simulink model "PMSM_Hall_model"  (R2025b)
settings: Solver=VariableStepAuto  StartTime=0.0  StopTime=10.0  RelTol=1e-3
values from neighbouring files (symbols this model uses):
  B = 0.0025    [PMSM_Hall_Model_script.m]
  Damping_viscous = 0.00012    [PMSM_Hall_Model_script.m]
  J = 4.5e-5    (= 4.5e-05)    [PMSM_Hall_Model_script.m]
  Ki_Id = omg_clc * R_s    (= 464.72)    [PMSM_Hall_Model_script.m]
  Ki_Iq = omg_clc * R_s    (= 464.72)    [PMSM_Hall_Model_script.m]
  Kp_Id = omg_clc * Ld    (= 22.608)    [PMSM_Hall_Model_script.m]
  Kp_Iq = omg_clc * Lq    (= 22.608)    [PMSM_Hall_Model_script.m]
  motor_polepairs = 7    [PMSM_Hall_Model_script.m]
  pwm_frequency = 20e3    (= 20000)    [PMSM_Hall_Model_script.m]
  x = 600    [PMSM_Hall_Model_script.m]
libraries: nesl_utility x9, slpidlib x5, fl_lib x5, mcbeeMathTransformLib x3, ee_lib x3, mcbcontrolslib x1, mcbsensorlessestimatorlib x1, mcbplantlib x1, autolibpmsmexterior x1, sdl_lib x1
settings Model: Creator=Surinova  LastModifiedBy=Surinova

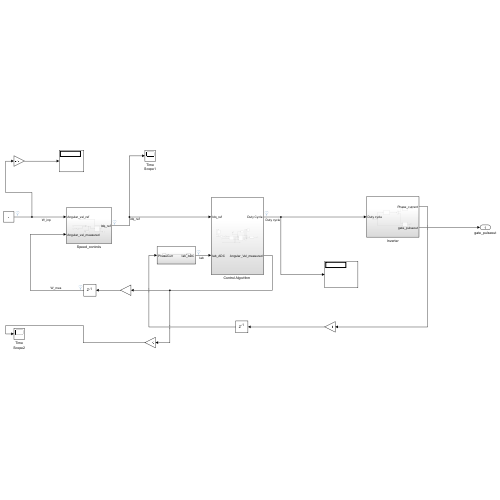
[thumbnail: Simulink's stored preview of the top-level diagram]
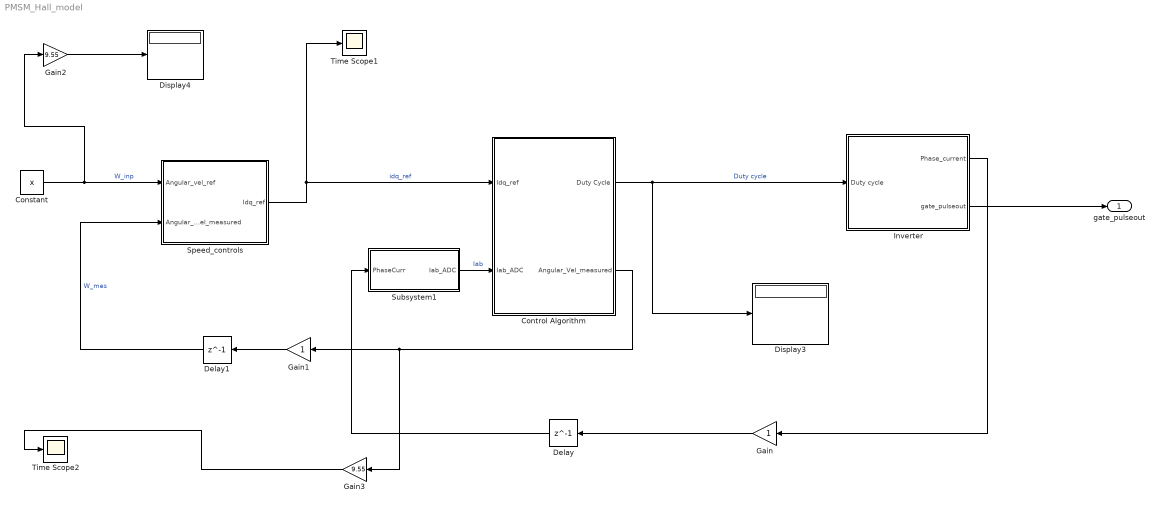
== system PMSM_Hall_model ==
  Constant : Constant  Value=x
  "Control Algorithm " : Subsystem
  Delay : Delay  DelayLength=1
  Delay1 : Delay  DelayLength=1
  Display3 : Display
  Display4 : Display
  Gain : Gain
  Gain1 : Gain
  Gain2 : Gain  Gain=9.55
  Gain3 : Gain  Gain=9.55
  Inverter : Subsystem
  Speed_controls : Subsystem
  Subsystem1 : Subsystem
  Time Scope1 : Scope
      settings: TimeUnits=Metric (based on Time Span)  ActiveDisplayYMinimum=-1278.396312713623  ActiveDisplayYMaximum=607.25992965698242  YLabel=Amplitude
  Time Scope2 : Scope
      settings: TimeUnits=Metric (based on Time Span)  ActiveDisplayYMinimum=-2551.3535904439232  ActiveDisplayYMaximum=7986.0366937033405  YLabel=Amplitude  DataLoggingVariableName=ScopeData5
  gate_pulseout : Outport
  wires:
  Speed_controls/1(Idq_ref) -> Time Scope1/1, "Control Algorithm "/1(Idq_ref)  "idq_ref"
  Delay/1 -> Subsystem1/1(PhaseCurr)
  "Control Algorithm "/2(Angular_Vel_measured) -> Gain1/1, Gain3/1
  Gain/1 -> Delay/1
  Delay1/1 -> Speed_controls/2(Angular_vel_measured)  "W_mes"
  Constant/1 -> Gain2/1, Speed_controls/1(Angular_vel_ref)  "W_inp"
  Subsystem1/1(Iab_ADC) -> "Control Algorithm "/2(Iab_ADC)  "Iab"
  Gain3/1 -> Time Scope2/1
  "Control Algorithm "/1(Duty Cycle) -> Inverter/1(Duty cycle), Display3/1  "Duty cycle"
  Inverter/1(Phase_current) -> Gain/1
  Gain2/1 -> Display4/1
  Inverter/2(gate_pulseout) -> gate_pulseout/1
  Gain1/1 -> Delay1/1

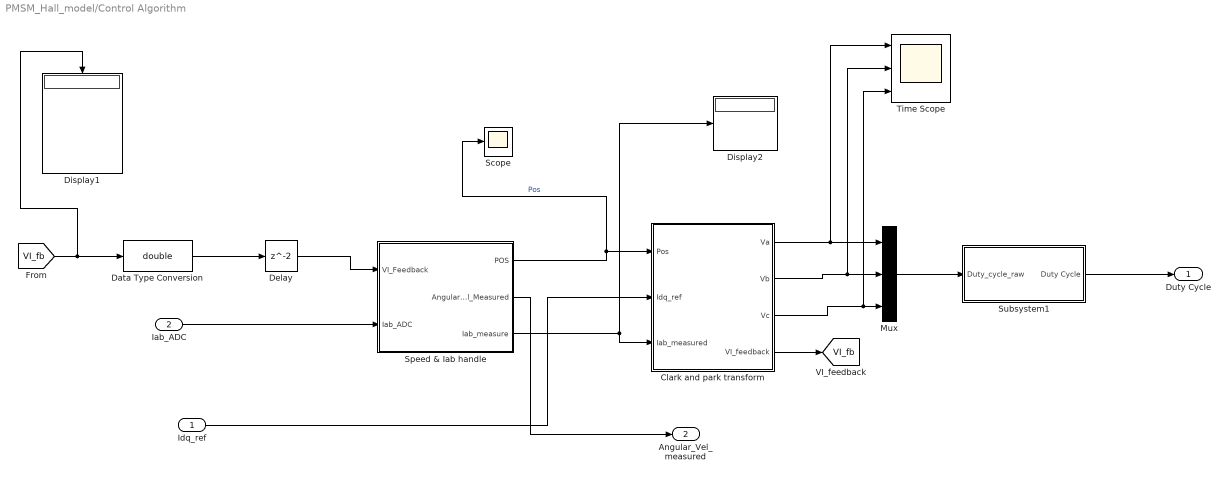
== system PMSM_Hall_model/Control Algorithm  ==
  Idq_ref : Inport
  Iab_ADC : Inport  Port=2
  Clark and park transform : Subsystem
  Data Type Conversion : DataTypeConversion  OutDataTypeStr=double  SaturateOnIntegerOverflow=off  RndMeth=Floor
  Delay : Delay
  Display1 : Display
  Display2 : Display
  Mux : Mux  Inputs=3
  Scope : Scope
      settings: ActiveDisplayYMinimum=-2.9858848726720835  ActiveDisplayYMaximum=10.141823403799465  DataLoggingVariableName=ScopeData4
  Speed & Iab handle : Subsystem
  Subsystem1 : Subsystem
  Time Scope : Scope  NumInputPorts=3
      settings: TimeUnits=Metric (based on Time Span)  ActiveDisplayYMinimum=-2.8960393222402327  ActiveDisplayYMaximum=4.8327650583252995  YLabel=Amplitude  DataLoggingVariableName=ScopeData2
  Duty Cycle : Outport
  Angular_Vel_measured : Outport  Port=2
  tag scope: VI_fb=global
  wires:
  Clark and park transform/4(VI_feedback) -> [VI_fb]
  Clark and park transform/3(Vc) -> Mux/3, Time Scope/3
  [VI_fb] -> Display1/1, Data Type Conversion/1
  Mux/1 -> Subsystem1/1(Duty_cycle_raw)
  Iab_ADC/1 -> Speed & Iab handle/2(Iab_ADC)
  Speed & Iab handle/3(Iab_measure) -> Clark and park transform/3(Iab_measured), Display2/1
  Clark and park transform/2(Vb) -> Mux/2, Time Scope/2
  Clark and park transform/1(Va) -> Time Scope/1, Mux/1
  Speed & Iab handle/2(Angular_Vel_Measured) -> Angular_Vel_measured/1
  Idq_ref/1 -> Clark and park transform/2(Idq_ref)
  Delay/1 -> Speed & Iab handle/1(VI_Feedback)
  Data Type Conversion/1 -> Delay/1
  Speed & Iab handle/1(POS) -> Scope/1, Clark and park transform/1(Pos)  "Pos"
  Subsystem1/1(Duty Cycle) -> Duty Cycle/1

== system PMSM_Hall_model/Inverter ==
  Duty cycle : Inport
  Codegen : Subsystem
  Simulation : Subsystem
  Subsystem2 : Subsystem
  Variant Sink : VariantSink  VariantControlMode=sim codegen switching  ShowConditionOnBlock=on  VariantControls={(codegen), (sim)}
  Phase_current : Outport
  gate_pulseout : Outport  Port=2
  wires:
  Duty cycle/1 -> Simulation/2(Duty_cycle), Subsystem2/1(Duty cycle)
  Subsystem2/1(Duty_cycle_6pulse) -> Variant Sink/1  "Gate_pulse"
  Simulation/1(Phase_current) -> Phase_current/1
  Variant Sink/2 -> Simulation/1(Gate_pulse)
  Variant Sink/1 -> Codegen/1(gate_pulse)
  Codegen/1(gate_pulseout) -> gate_pulseout/1

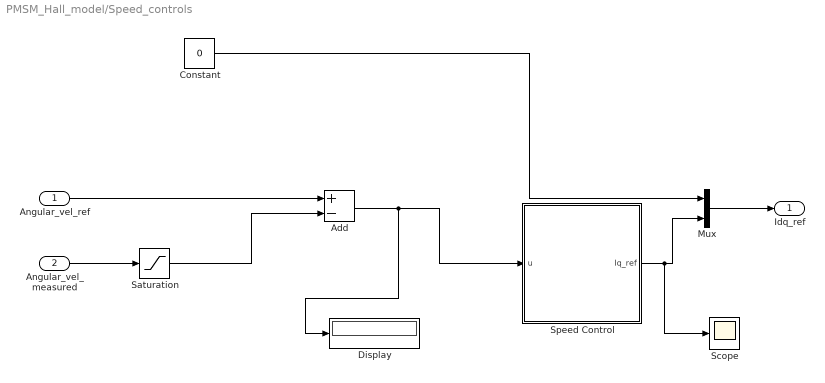
== system PMSM_Hall_model/Speed_controls ==
  Angular_vel_ref : Inport
  Angular_vel_measured : Inport  Port=2
  Add : Sum  Inputs=+-
  Constant : Constant  Value=0
  Display : Display
  Mux : Mux  Inputs=2
  Saturation : Saturate  UpperLimit=600  LowerLimit=-600
  Scope : Scope
      settings: ActiveDisplayYMinimum=-1  ActiveDisplayYMaximum=1  DataLoggingVariableName=ScopeData3
  Speed Control : Subsystem
  Idq_ref : Outport  PortDimensions=2
  wires:
  Angular_vel_measured/1 -> Saturation/1
  Add/1 -> Display/1, Speed Control/1(u)
  Mux/1 -> Idq_ref/1
  Speed Control/1(Iq_ref) -> Scope/1, Mux/2
  Constant/1 -> Mux/1
  Angular_vel_ref/1 -> Add/1
  Saturation/1 -> Add/2

== system PMSM_Hall_model/Subsystem1 ==
  PhaseCurr : Inport
  Iab_ADC : Outport
  wires:
  PhaseCurr/1 -> Iab_ADC/1

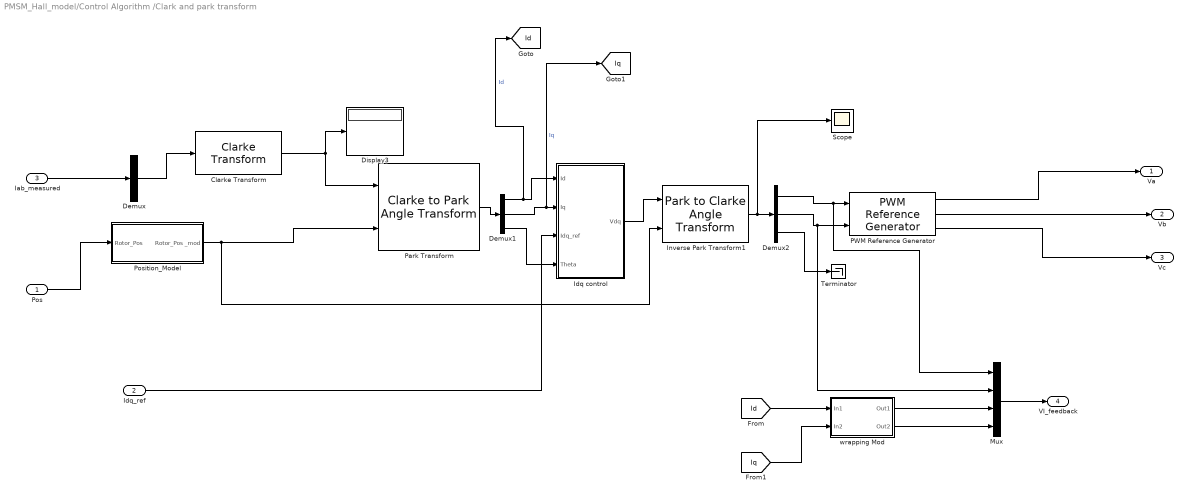
== system PMSM_Hall_model/Control Algorithm /Clark and park transform ==
  Pos : Inport
  Idq_ref : Inport  Port=2
  Iab_measured : Inport  Port=3
  Clarke Transform : mcbeeMathTransformLib/Clarke Transform  VariantControl=Variant2  PowerInvariant=off  UseWithEmbedded=on  PhaseInput=Three inputs
      settings: LibrarySourceBlock=mcblib/Controls/Math Transforms/Clarke Transform
  Demux : Demux  Outputs=1
  Demux1 : Demux  Outputs=3
  Demux2 : Demux  Outputs=3
  Display3 : Display
  Idq control : Subsystem
  Inverse Park Transform1 : mcbeeMathTransformLib/Park to Clarke Angle Transform  AxisAlignment=D-axis  UseWithEmbedded=on  PhaseInput=Three inputs  ThetaInput=Electrical position  AngleInput=Radians  N_points=1024
      settings: LibrarySourceBlock=mcbhdllib/Controls/Math Transforms/Inverse Park Transform
  Mux : Mux
  PWM Reference Generator : mcbcontrolslib/PWM Reference Generator  inSignal=Valphabeta  modType=SVM: space vector modulation
      settings: LibrarySourceBlock=mcbhdllib/Controls/Math Transforms/PWM Reference Generator
  Park Transform : mcbeeMathTransformLib/Clarke to Park Angle Transform  AxisAlignment=D-axis  UseWithEmbedded=on  PhaseInput=Three inputs  ThetaInput=Electrical position  AngleInput=Radians  N_points=1024
      settings: LibrarySourceBlock=mcblib/Controls/Math Transforms/Park Transform
  Position_Model : Subsystem
  Scope : Scope
      settings: ActiveDisplayYMinimum=-1.6231207105132253  ActiveDisplayYMaximum=1.9168476700347847  DataLoggingVariableName=ScopeData9
  Terminator : Terminator
  wrapping Mod : Subsystem
  Va : Outport
  Vb : Outport  Port=2
  Vc : Outport  Port=3
  VI_feedback : Outport  Port=4
  tag scope: Id=global, Iq=global
  wires:
  Clarke Transform/1 -> Park Transform/1, Display3/1
  Demux/1 -> Clarke Transform/1
  PWM Reference Generator/1 -> Va/1
  PWM Reference Generator/2 -> Vb/1
  PWM Reference Generator/3 -> Vc/1
  Idq_ref/1 -> Idq control/3(Idq_ref)
  Mux/1 -> VI_feedback/1
  Iab_measured/1 -> Demux/1
  wrapping Mod/1(Out1) -> Mux/3
  wrapping Mod/2(Out2) -> Mux/4
  Pos/1 -> Position_Model/1(Rotor_Pos)
  Position_Model/1(Rotor_Pos _mod) -> Inverse Park Transform1/2, Park Transform/2
  Park Transform/1 -> Demux1/1
  Demux1/2 -> [Iq], Idq control/2(Iq)  "Iq"
  Demux1/3 -> Idq control/4(Theta)
  Idq control/1(Vdq) -> Inverse Park Transform1/1
  Inverse Park Transform1/1 -> Scope/1, Demux2/1
  Demux2/1 -> Mux/1, PWM Reference Generator/1
  Demux2/2 -> Mux/2, PWM Reference Generator/2
  Demux2/3 -> Terminator/1
  Demux1/1 -> [Id], Idq control/1(Id)  "Id"
  [Id] -> wrapping Mod/1(In1)
  [Iq] -> wrapping Mod/2(In2)

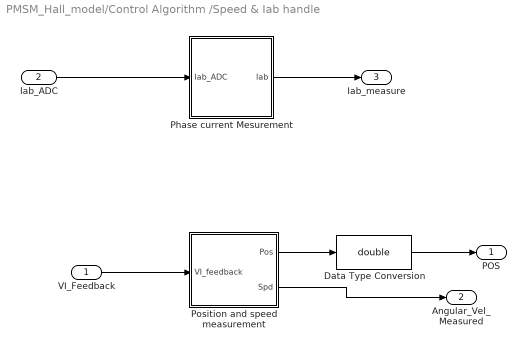
== system PMSM_Hall_model/Control Algorithm /Speed & Iab handle ==
  VI_Feedback : Inport
  Iab_ADC : Inport  Port=2
  Data Type Conversion : DataTypeConversion  OutDataTypeStr=double  SaturateOnIntegerOverflow=off  RndMeth=Floor
  Phase current Mesurement : Subsystem
  Position and speed measurement : Subsystem
  POS : Outport
  Angular_Vel_Measured : Outport  Port=2
  Iab_measure : Outport  Port=3
  wires:
  VI_Feedback/1 -> Position and speed measurement/1(VI_feedback)
  Position and speed measurement/1(Pos) -> Data Type Conversion/1
  Position and speed measurement/2(Spd) -> Angular_Vel_Measured/1
  Iab_ADC/1 -> Phase current Mesurement/1(Iab_ADC)
  Phase current Mesurement/1(Iab) -> Iab_measure/1
  Data Type Conversion/1 -> POS/1

== system PMSM_Hall_model/Control Algorithm /Subsystem1 ==
  Duty_cycle_raw : Inport
  Add : Sum
  Constant : Constant  Value=1.45
  Gain : Gain  Gain=1/3
  Duty Cycle : Outport
  wires:
  Constant/1 -> Add/2
  Add/1 -> Gain/1
  Duty_cycle_raw/1 -> Add/1
  Gain/1 -> Duty Cycle/1

== system PMSM_Hall_model/Inverter/Codegen ==
  note: Hardware region
      | gate pulse fed todriver via controller
  gate_pulse : Inport
  gate_pulseout : Outport
  wires:
  gate_pulse/1 -> gate_pulseout/1

== system PMSM_Hall_model/Inverter/Simulation ==
  Gate_pulse : Inport
  Duty_cycle : Inport  Port=2
  Inverter&motor_Plant_model : Subsystem
  Scope : Scope  NumInputPorts=2
      settings: ActiveDisplayYMinimum=-225.10774527747819  ActiveDisplayYMaximum=225.10294010409339  DataLoggingVariableName=ScopeData7
  Simscape_Plantmodel : Subsystem
  Time Scope : Scope
      settings: TimeUnits=Metric (based on Time Span)  ActiveDisplayYMinimum=-4.9999999999993694  ActiveDisplayYMaximum=44.999999999994344  YLabel=Amplitude
  Phase_current : Outport
  wires:
  Inverter&motor_Plant_model/1(Electrical Pos) -> Scope/1  "Ele_Pos"
  Simscape_Plantmodel/1(Angular_vel_measured) -> Time Scope/1  "W_fb_sim"
  Inverter&motor_Plant_model/3(Motor_trq) -> Scope/2  "Motor_rpm"
  Inverter&motor_Plant_model/2(PhaseCurrent) -> Phase_current/1  "Phase_current"
  Gate_pulse/1 -> Simscape_Plantmodel/1(Duty Cycle_6pulse)
  Duty_cycle/1 -> Inverter&motor_Plant_model/1(Duty_cycle)

== system PMSM_Hall_model/Inverter/Subsystem2 ==
  Duty cycle : Inport
  Demux : Demux  Outputs=3
  Demux1 : Demux  Outputs=3
  Gate_pulse : Scope  NumInputPorts=6
      settings: TimeUnits=Metric (based on Time Span)  ActiveDisplayYMinimum=-0.2043367875881458  ActiveDisplayYMaximum=0.55931759444230922  YLabel=Amplitude  DataLoggingVariableName=ScopeData10
  Mux : Mux  Inputs=6
  Subsystem : Subsystem
  Duty_cycle_6pulse : Outport
  wires:
  Demux1/1 -> Mux/2, Gate_pulse/4  "GA_L"
  Demux/2 -> Mux/3, Gate_pulse/2  "GB_H"
  Duty cycle/1 -> Demux/1, Subsystem/1(Duty Cycle)
  Demux/1 -> Mux/1, Gate_pulse/1  "GA_H"
  Subsystem/1(Gate_Lowside) -> Demux1/1
  Demux1/2 -> Mux/4, Gate_pulse/5  "GB_L"
  Demux1/3 -> Mux/6, Gate_pulse/6  "GC_L"
  Demux/3 -> Mux/5, Gate_pulse/3  "GC_H"
  Mux/1 -> Duty_cycle_6pulse/1

== system PMSM_Hall_model/Speed_controls/Speed Control ==
  u : Inport
  PID Controller : slpidlib/PID Controller  Controller=PI  Form=Parallel  TimeDomain=Continuous-time  UseExternalTs=off  SampleTime=-1  IntegratorMethod=Forward Euler  FilterMethod=Forward Euler  ControllerParametersSource=internal  P=1  I=0  UseKiTs=off  D=0  UseExternalDerivativeSource=off  N=100  UseFilter=on  TunerSelectOption=Transfer Function Based (PID Tuner App)  InitialConditionSource=internal  InitialConditionForIntegrator=0  InitialConditionForFilter=0  DifferentiatorICPrevScaledInput=0  ExternalReset=none  TrackingMode=off  Kt=1  LimitOutput=off  SatLimitsSource=internal  UpperSaturationLimit=inf  LowerSaturationLimit=-inf  LinearizeAsGain=on  AntiWindupMode=none  Kb=1  LimitIntegrator=off  UpperIntegratorSaturationLimit=inf  LowerIntegratorSaturationLimit=-inf  POutMin=[]  POutMax=[]  IOutMin=[]  IOutMax=[]  DOutMin=[]  DOutMax=[]  NOutMin=[]  NOutMax=[]  SumOutMin=[]  SumOutMax=[]  SaturationOutMin=[]  SaturationOutMax=[]  PParamMin=[]  PParamMax=[]  IParamMin=[]  IParamMax=[]  DParamMin=[]  DParamMax=[]  NParamMin=[]  NParamMax=[]  KbParamMin=[]  KbParamMax=[]  KtParamMin=[]  KtParamMax=[]  KbOutMin=[]  KbOutMax=[]  KtOutMin=[]  KtOutMax=[]  IntegratorOutMin=[]  IntegratorOutMax=[]  FilterOutMin=[]  FilterOutMax=[]  SumI1OutMin=[]  SumI1OutMax=[]  SumI2OutMin=[]  SumI2OutMax=[]  SumI3OutMin=[]  SumI3OutMax=[]  SumI4OutMin=[]  SumI4OutMax=[]  SumDOutMin=[]  SumDOutMax=[]  DifferentiatorOutMin=[]  DifferentiatorOutMax=[]  FilterDiffOutCoefMin=[]  FilterDiffOutCoefMax=[]  ReciprocalOutMin=[]  ReciprocalOutMax=[]  SumDenOutMin=[]  SumDenOutMax=[]  SumNumOutMin=[]  SumNumOutMax=[]  DivideOutMin=[]  DivideOutMax=[]  UdiffTsProdOutMin=[]  UdiffTsProdOutMax=[]  NTsProdOutMin=[]  NTsProdOutMax=[]  UintegralTsProdOutMin=[]  UintegralTsProdOutMax=[]  UngainTsProdOutMin=[]  UngainTsProdOutMax=[]  ClampingZeroOutDataTypeStr=Inherit: Inherit via back propagation  ClampingZeroOutMin=[]  ClampingZeroOutMax=[]  FilterDenConstantOutDataTypeStr=Inherit: Inherit via back propagation  FilterDenConstantOutMin=[]  FilterDenConstantOutMax=[]  PCopyOutDataTypeStr=Inherit: Inherit via back propagation  PCopyOutMin=[]  PCopyOutMax=[]  NCopyOutDataTypeStr=Inherit: Inherit via back propagation  NCopyOutMin=[]  NCopyOutMax=[]  IntegratorContinuousStateAttributes=''  IntegratorStateMustResolveToSignalObject=off  IntegratorRTWStateStorageClass=Auto  FilterContinuousStateAttributes=''  FilterStateMustResolveToSignalObject=off  FilterRTWStateStorageClass=Auto  ParallelPVariant=InternalParameters  IdealPVariant=Disabled  IVariant=InternalParameters  DVariant=Disabled  IntegratorVariant=Continuous  SatVariant=Disabled  AWVariant=Passthrough  PCopyVariant=Disabled  TRVariant=Disabled  FdbkBlocksVariant=Forward  IdealPFdbkVariant=Disabled  SatFdbkVariant=Disabled  DerivativeFilterVariant=Disabled  NVariant=Disabled  NCopyVariant=Disabled_SignalSpec  FilterICVariant=Disabled  IntegratorICVariant=InternalICs  ExternalResetVariant=Disabled  TRSumVariant=Passthrough  SumFdbkVariant=Disabled  SumVariant=Sum_PI  TsampFilterVariant=InternalTs  TsampNgainVariant=Passthrough  TsampIntegralVariant=Disabled_SignalSpec  ExternalSaturationOutDataTypeStr=Inherit: Same as second input  DerivativeSourceVariant=Disabled  PreIntVariant=InternalPreInt
  Iq_ref : Outport
  wires:
  u/1 -> PID Controller/1
  PID Controller/1 -> Iq_ref/1

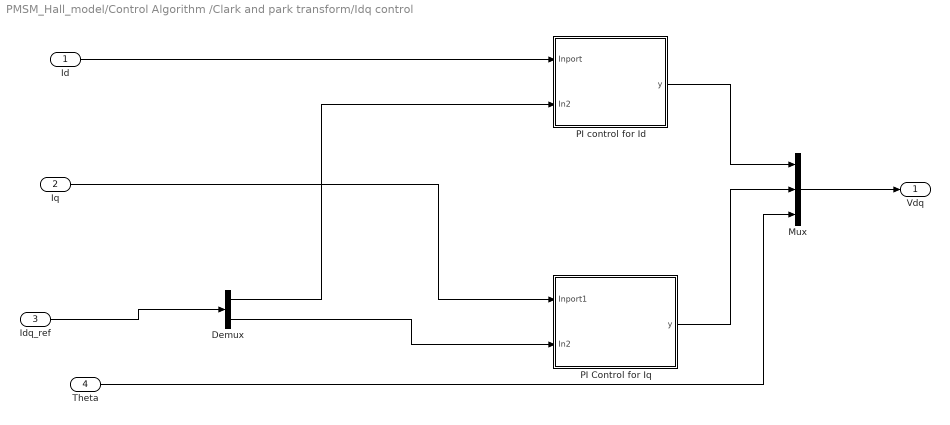
== system PMSM_Hall_model/Control Algorithm /Clark and park transform/Idq control ==
  Id : Inport
  Iq : Inport  Port=2
  Idq_ref : Inport  Port=3
  Theta : Inport  Port=4
  Demux : Demux  Outputs=2
  Mux : Mux  Inputs=3
  PI Control for Iq : Subsystem
  PI control for Id : Subsystem
  Vdq : Outport
  wires:
  Idq_ref/1 -> Demux/1
  Id/1 -> PI control for Id/1(Inport)
  Iq/1 -> PI Control for Iq/1(Inport1)
  Demux/1 -> PI control for Id/2(In2)
  Demux/2 -> PI Control for Iq/2(In2)
  PI control for Id/1(y) -> Mux/1
  PI Control for Iq/1(y) -> Mux/2
  Mux/1 -> Vdq/1
  Theta/1 -> Mux/3

== system PMSM_Hall_model/Control Algorithm /Clark and park transform/Position_Model ==
  Rotor_Pos : Inport
  Constant : Constant  Value=2*3.141
  Data Type Conversion1 : DataTypeConversion  OutDataTypeStr=double  ConvertRealWorld=Stored Integer (SI)  RndMeth=Floor
  Display : Display
  Mod : Math  Operator=mod
  Rotor_Pos _mod : Outport
  wires:
  Mod/1 -> Data Type Conversion1/1
  Constant/1 -> Mod/2
  Rotor_Pos/1 -> Mod/1  "Eps"
  Data Type Conversion1/1 -> Rotor_Pos _mod/1, Display/1

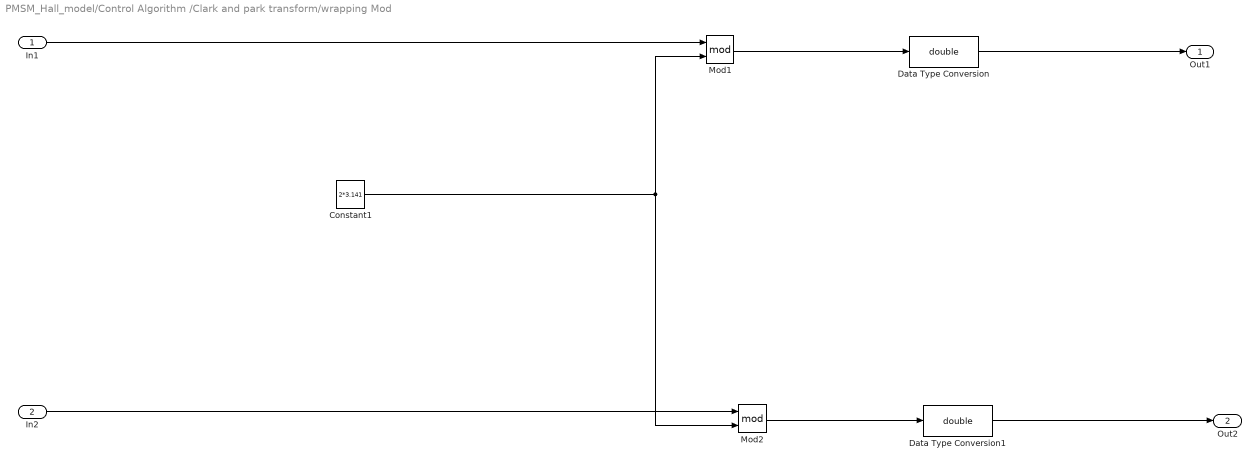
== system PMSM_Hall_model/Control Algorithm /Clark and park transform/wrapping Mod ==
  In1 : Inport
  In2 : Inport  Port=2
  Constant1 : Constant  Value=2*3.141
  Data Type Conversion : DataTypeConversion  OutDataTypeStr=double  SaturateOnIntegerOverflow=off  RndMeth=Floor
  Data Type Conversion1 : DataTypeConversion  OutDataTypeStr=double  SaturateOnIntegerOverflow=off  RndMeth=Floor
  Mod1 : Math  Operator=mod
  Mod2 : Math  Operator=mod
  Out1 : Outport
  Out2 : Outport  Port=2
  wires:
  Constant1/1 -> Mod2/2, Mod1/2
  In1/1 -> Mod1/1
  In2/1 -> Mod2/1
  Mod2/1 -> Data Type Conversion1/1
  Mod1/1 -> Data Type Conversion/1
  Data Type Conversion/1 -> Out1/1
  Data Type Conversion1/1 -> Out2/1

== system PMSM_Hall_model/Control Algorithm /Speed & Iab handle/Phase current Mesurement ==
  Iab_ADC : Inport
  Data Type Conversion : DataTypeConversion  SaturateOnIntegerOverflow=off  RndMeth=Floor
  Iab : Outport
  wires:
  Data Type Conversion/1 -> Iab/1
  Iab_ADC/1 -> Data Type Conversion/1

== system PMSM_Hall_model/Control Algorithm /Speed & Iab handle/Position and speed measurement ==
  VI_feedback : Inport
  Demux : Demux
  Extended EMF Observer : mcbsensorlessestimatorlib/Extended EMF Observer  ParameterBusInput=off  InputUnit=SI unit  PosOut=Electrical position  BlkSampleTime=1/pwm_frequency  StatorResistance=R_s  StatorDaxisInductance=Ld  StatorQaxisInductance=Lq  MaxApplicationSpeed=6000  PolePairs=motor_polepairs  MaxStatorVoltage=48  MaxStatorCurrent=20  Alpha=1  EEMFCutoffFreq=7500  Kp=250  Ki=100000  N_points=1024  SpeedCutoffFreq=15  PositionUnit=Radians  PositionDataType=single  SpeedUnit=Radians/sec  PerUnitSpeed=6000  SpeedDataType=single  TableDatatype=single
      settings: LibrarySourceBlock=mcblib/Sensorless Estimators/Extended EMF Observer
  Pos : Outport
  Spd : Outport  Port=2
  wires:
  Demux/1 -> Extended EMF Observer/1
  Demux/2 -> Extended EMF Observer/2
  Extended EMF Observer/1 -> Pos/1
  VI_feedback/1 -> Demux/1
  Demux/3 -> Extended EMF Observer/3
  Demux/4 -> Extended EMF Observer/4
  Extended EMF Observer/2 -> Spd/1

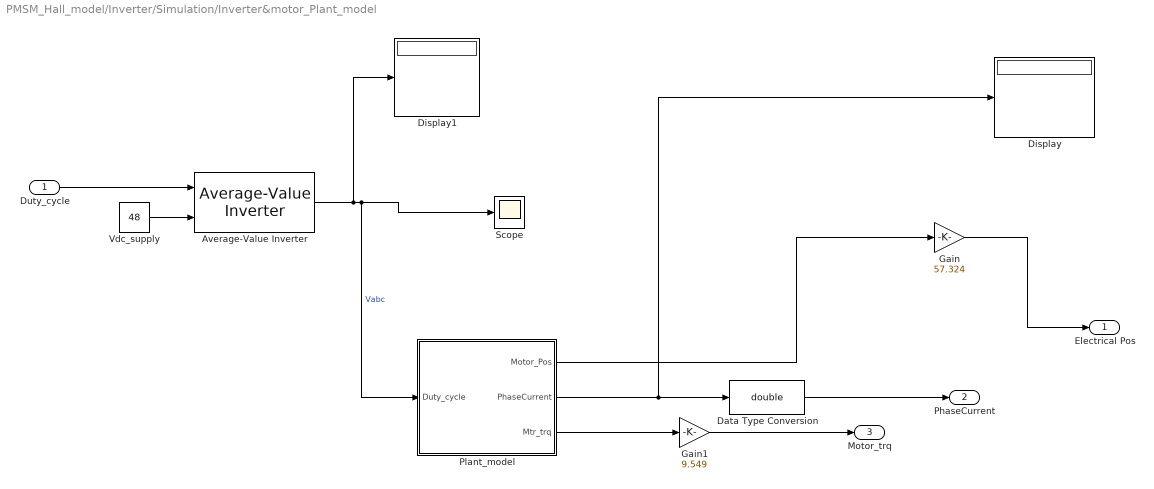
== system PMSM_Hall_model/Inverter/Simulation/Inverter&motor_Plant_model ==
  Duty_cycle : Inport
  Average-Value Inverter : mcbplantlib/Average-Value Inverter
      settings: LibrarySourceBlock=mcblib/Electrical Systems/Inverters/Average-Value Inverter
  Data Type Conversion : DataTypeConversion  OutDataTypeStr=double  RndMeth=Floor
  Display : Display
  Display1 : Display
  Gain : Gain  Gain=57.324
  Gain1 : Gain  Gain=9.549
  Plant_model : Subsystem
  Scope : Scope
      settings: ActiveDisplayYMinimum=-32.6598622851583  ActiveDisplayYMaximum=32.659861680116862  DataLoggingVariableName=ScopeData8
  Vdc_supply : Constant  Value=48
  Electrical Pos : Outport
  PhaseCurrent : Outport  Port=2
  Motor_trq : Outport  Port=3
  wires:
  Plant_model/2(PhaseCurrent) -> Display/1, Data Type Conversion/1
  Data Type Conversion/1 -> PhaseCurrent/1
  Plant_model/3(Mtr_trq) -> Gain1/1
  Duty_cycle/1 -> Average-Value Inverter/1
  Average-Value Inverter/1 -> Display1/1, Scope/1, Plant_model/1(Duty_cycle)  "Vabc"
  Vdc_supply/1 -> Average-Value Inverter/2
  Plant_model/1(Motor_Pos) -> Gain/1
  Gain/1 -> Electrical Pos/1
  Gain1/1 -> Motor_trq/1

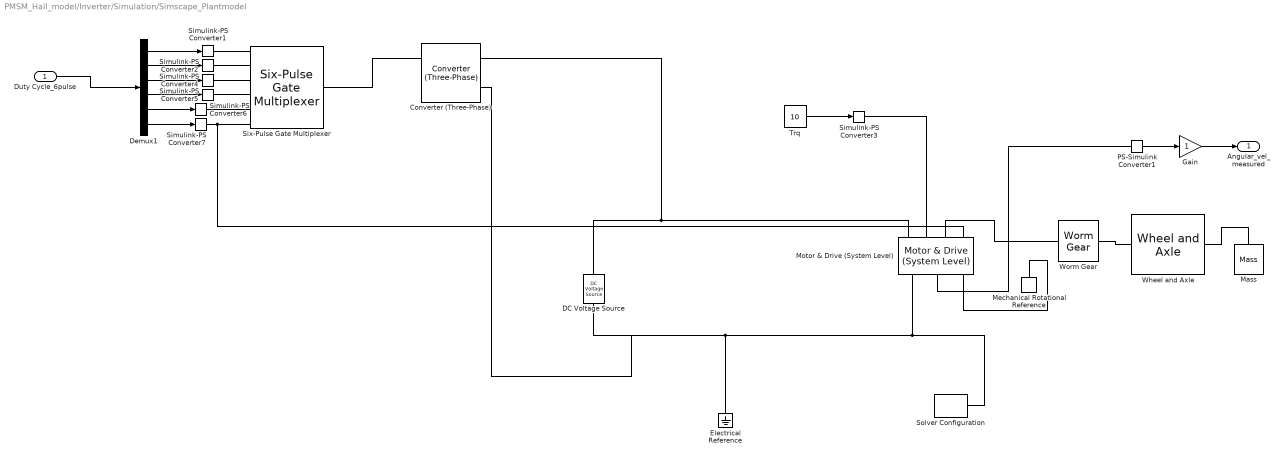
== system PMSM_Hall_model/Inverter/Simulation/Simscape_Plantmodel ==
  Duty Cycle_6pulse : Inport
  Converter (Three-Phase) : ee_lib/Semiconductors & Converters/Converters/Converter (Three-Phase)  port_option=ee.enum.threePhasePort.composite  fidelity_option=ee.enum.converters.fidelity.detailed  device_type=ee.enum.converters.switchingdevice.ideal  showThermalPort=false  K=0  Vth=6 V  Vgt=1 V  Vgt_off=-1 V  Ih=1 A  Vf=0.8 V  Ron=0.001 Ohm  Rds=0.001 Ohm  Goff=1e-6 1/Ohm  Eon_scalar=22.86e-3 J  Eoff_scalar=17.14e-3 J  Eoff_natural_commutation=10e-3 J  Voff=300 V  Iout_scalar=600 A  onCurrentMeasDelay=0 s  useCurrentFromPreviousCycle=false  useVoltageFromPreviousCycle=false  diode_param=ee.enum.converters.protectiondiode.none  diode_Vf=0.8 V  diode_Ron=0.001 Ohm  diode_Goff=1e-5 1/Ohm  diode_C=50 nF  diode_iRM=-235 A  diode_iF=300 A  diode_idot=-50 A/us  diode_trr_param=ee.enum.converters.diodetrr.trr_factor  diode_trr_factor=3  diode_trr=15 us  diode_Qrr=1500 s*uA  diode_rec_loss_model=ee.enum.diode.reverseRecoveryModel.fixed  diode_ErecVal=0 J  diode_scaleWithIandV=false  diode_ErecMat=zeros(2, 3) J  diode_TjrecVec=[298.15, 398.15] K  diode_IfrecVec=[.1, 1, 10] A  diode_IrecVal=10 A  diode_VrecVal=10 V  diode_tFilter=1 / 1000 / 100 s  thermal_network_parameterization=ee.enum.thermalNetworkTopology.external  Rth=[.08, .5] K/W  Rth_Cauer=[.08, .1, .5] K/W  Rth_Foster=[.08, .14, .22, .16] K/W  thermal_mass_parameterization=ee.enum.thermalNetwork.timeconstant  thermal_mass=[.01, .5] J/K  thermal_mass_Cauer=[.01, .1, .5] J/K  thermal_mass_Foster=[.001, .005, .05, .5] J/K  thermal_time_constant=[.001, .2] s  thermal_time_constant_Cauer=[.001, .1, .2] s  thermal_time_constant_Foster=[7e-05, .0007, .01, .08] s  thermal_mass_initial_temperatures=[25, 25] degC  thermal_mass_initial_temperatures_Cauer=[25, 25, 25] degC  junction_thermal_mass=0.01 J/K  Tvec_initial_Foster=[25, 25, 25, 25] degC  snubber_type=ee.enum.converters.snubber.exclude  Cs=1e-7 F  Rs=0.1 Ohm  Vce_loss=[0, 150, 300] V
  DC Voltage Source : fl_lib/Electrical/Electrical Sources/DC Voltage Source  v0=48 V
  Demux1 : Demux  Outputs=6
  Electrical Reference : fl_lib/Electrical/Electrical Elements/Electrical Reference
  Gain : Gain
  Mass : fl_lib/Mechanical/Translational Elements/Mass  mass=10 g  num_ports=foundation.enum.numPorts2.one  v_specify=on  v_priority=High  v=0 m/s  v_nominal_specify=off  v_nominal_value=1  v_nominal_unit=m/s  f_specify=off  f_priority=None  f=0 N  f_nominal_specify=off  f_nominal_value=1  f_nominal_unit=N
  Mechanical Rotational Reference : fl_lib/Mechanical/Rotational Elements/Mechanical Rotational Reference
  Motor & Drive (System Level) : ee_lib/Electromechanical/Motor & Drive (System Level)  torque_speed_param=ee.enum.electromech.envelope.torque_power  overtorque_param=ee.enum.electromech.overtorque.no  T_t=Torque N*m  T_t_intermittent=[.36, .32, .28, 0] N*m  T_t_2D=Torque N*m  T_t_intermittent_2D=[.36, .36, .36; .32, .32, .32; .28, .28, .28; 0, 0, 0] N*m  w_t=speed rpm  vdc_t=Vdc V  torque_max=0.1 N*m  power_max=30 W  torque_max_intermittent=0.4 N*m  power_max_intermittent=120 W  time_overtorque=30 s  time_recover=60 s  Tc=Kv s  EnableSwitch=true  losses_param=1  eff=85  w_eff=3750 rpm  T_eff=0.08 N*m  Piron=0 W  Pbase=0 W  w_eff_vec=[-8000, -4000, 0, 4000, 8000] rpm  T_eff_vec=[0, .03, .06, .09] N*m  v_eff_vec=[22, 35, 50] V  losses_mat=[1.49, 1.67, 2.21, 3.1; .42, .69, 1.14, 2.03; .06, .24, .78, 1.68; .42, .69, 1.14, 2.03; 1.49, 1.67, 2.21, 3.1] W  efficiency_mat=[95, 95, 95, 95; 95, 95, 95, 95; 95, 95, 95, 95; 95, 95, 95, 95; 95, 95, 95, 95]  losses_mat_3D=ones(5, 4, 3) W  efficiency_mat_3D=95 * ones(5, 4, 3)  Res=R_s Ohm  J=J kg*m^2  lam=B N*m*s/rad  speed0=0 rpm  faulted_specify=off  faulted_priority=None  faulted=0  faulted_nominal_specify=off  faulted_nominal_value=1  faulted_nominal_unit=1  isSwitchedOff_specify=off  isSwitchedOff_priority=None  isSwitchedOff=0  isSwitchedOff_nominal_specify=off  isSwitchedOff_nominal_value=1  isSwitchedOff_nominal_unit=1  torqueLimitContinuous_specify=off  torqueLimitContinuous_priority=None  torqueLimitContinuous=0 N*m  torqueLimitContinuous_nominal_specify=off  torqueLimitContinuous_nominal_value=1  torqueLimitContinuous_nominal_unit=N*m  alpha=3.93e-3 1/K  Tmeas=25 degC  Tmeas2=125 degC  losses_mat_T2=[1.49, 1.74, 2.49, 3.74; .42, .67, 1.42, 2.67; .06, .31, 1.06, 2.31; .42, .67, 1.42, 2.67; 1.49, 1.74, 2.49, 3.74] W  efficiency_mat_T2=[95, 95, 95, 95; 95, 95, 95, 95; 95, 95, 95, 95; 95, 95, 95, 95; 95, 95, 95, 95]  losses_mat_3D_T2=ones(5, 4, 3) W  efficiency_mat_3D_T2=95 * ones(5, 4, 3)  thermal_mass=100 J/K  initial_temperature=25 degC
      settings: InternalSimscapePortConfiguration="{\"Bottom\":[],\"Left\":[{\"id\":\"Vp\",\"label\":\"+\",\"type\":\"foundation.electrical.electrical\"},{\"id\":\"Tr\",\"label\":\"Tr\",\"type\":\"input\"},{\"id\":\"R\",\"label\":\"R\",\"type\":\"foundation.mechanical.rotational.rotational\"},{\"id\":\"F\",\"label\":\"OFF\",\"type\":\"input\"}],\"Right\":[{\"id\":\"Vm\",\"label\":\"-\",\"type\":\"foundation.electrical.electrical\"},{\"id\":\"Omega\",\"label\":\"w\",\"type\":\"output\"},{\"id\":\"C\",\"label\":\"C\",\"type\":\"foundation.mechanical.rotational.rotational\"}],\"Top\":[]}"
  PS-Simulink Converter1 : nesl_utility/PS-Simulink Converter  PhysicalDomain=network_engine_domain  SubClassName=ps_output  LeftPortType=input  RightPortType=output  PseudoPeriodic=off  Frequencies=[]  VectorFormat=inherit  Unit=rad/s  AffineConversion=off
  Simulink-PS Converter{1..2,4..7} (6 alike) : nesl_utility/Simulink-PS Converter  PhysicalDomain=network_engine_domain  SubClassName=ps_input  LeftPortType=input  RightPortType=output  PseudoPeriodic=off  Frequencies=[]  NoiseDistribution=none  NoiseParameters=[]  Unit=V  AffineConversion=off  FilteringAndDerivatives=provide  SimscapeFilterOrder=1  InputFilterTimeConstant=0.001  UdotUserProvided=0
  Simulink-PS Converter3 : nesl_utility/Simulink-PS Converter  PhysicalDomain=network_engine_domain  SubClassName=ps_input  LeftPortType=input  RightPortType=output  PseudoPeriodic=off  Frequencies=[]  NoiseDistribution=none  NoiseParameters=[]  Unit=N*m  AffineConversion=off  FilteringAndDerivatives=provide  SimscapeFilterOrder=1  InputFilterTimeConstant=0.001  UdotUserProvided=0
  Six-Pulse Gate Multiplexer : ee_lib/Semiconductors & Converters/Converters/Six-Pulse Gate Multiplexer  port_option=ee.enum.controlport.ps
  Solver Configuration : nesl_utility/Solver Configuration  PhysicalDomain=network_engine_domain  SubClassName=solver  LeftPortType=input  RightPortType=generic  Tones=[]  Harmonics=[]  SimulateNoise=off  Profile=off  UseLocalSampling=off  EnableSwitchedLinearOptims=on  FrequencyDomain=off  UseCCode=off  RelTol=0.001  AbsTol=0.001  MinStep=1e-09  ToWorkspace=off  RevertToSquareIcSolve=off  NumHomotopyIterations=100  PhasorMode=off  PhasorModeNumHarmonics=1  ConsistencySolver=NEWTON_XTOL_AFTER_FTOL  IndexReductionMethod=DerivativeReplacement  DoDC=on  ResidualTolerance=1e-09  ConsistencyTolSource=GLOBAL  ConsistencyAbsTol=0.001  ConsistencyRelTol=0.001  ConsistencyTolFactor=0.001  UseLocalSolver=off  LocalSolverChoice=NE_BACKWARD_EULER_ADVANCER  ResolveIndetEquations=on  FunctionEvalNumThread=1  LocalSolverSampleTime=0.001  DoFixedCost=off  MaxNonlinIter=3  MaxModeIter=2  ComputeImpulses=off  ImpulseIterations=2  LinearAlgebra=auto  LinearAlgebraNumThread=0  EquationFormulation=NE_TIME_EF  DelaysMemoryBudget=1024  AutomaticFiltering=off  FilteringTimeConstant=0.001  PartitionStorageMethod=AS_NEEDED  PartitionMemoryBudget=1024  PartitionMethod=ROBUST  MultibodyUseLocalSolver=on  MultibodyLocalSolverChoice=ODE1  MultibodyLocalSolverSampleTime=0.001
  Trq : Constant  Value=10
  Wheel and Axle : fl_lib/Mechanical/Mechanisms/Wheel and Axle  R=0.05 m  or=foundation.enum.DriveOrientation.Positive  t_specify=off  t_priority=None  t=0 N*m  t_nominal_specify=off  t_nominal_value=1  t_nominal_unit=N*m  f_specify=off  f_priority=None  f=0 N  f_nominal_specify=off  f_nominal_value=1  f_nominal_unit=N
  Worm Gear : sdl_lib/Gears/Worm Gear  ratio=25  thread_type=sdl.enum.handedness.right  friction_model=sdl.enum.gear_friction.none  friction_parameterization=sdl.enum.efficiency_geometry.geometry  pr_ang=17.5 deg  lead_ang=20 deg  fr_coeff=0.08  eff_wg=0.74  eff_gw=0.65  temperature_TLU=[280, 300, 320] K  efficiency_wg_TLU=[.75, .65, .6]  efficiency_gw_TLU=[.5, .45, .4]  pwr_thr=0.001 W  mu_visc=[0, 0] N*m*s/rad  thermal_mass=50 J/K  temperature_specify=off  temperature_priority=High  temperature=300 K  temperature_nominal_specify=off  temperature_nominal_value=1  temperature_nominal_unit=K
      settings: InternalSimscapePortConfiguration="{\"Bottom\":[],\"Left\":[{\"id\":\"W\",\"label\":\"W\",\"type\":\"foundation.mechanical.rotational.rotational\"}],\"Right\":[{\"id\":\"G\",\"label\":\"G\",\"type\":\"foundation.mechanical.rotational.rotational\"}],\"Top\":[]}"
  Angular_vel_measured : Outport
  wires:
  PS-Simulink Converter1/1 -> Gain/1
  Trq/1 -> Simulink-PS Converter3/1
  Duty Cycle_6pulse/1 -> Demux1/1
  Demux1/1 -> Simulink-PS Converter1/1
  Demux1/2 -> Simulink-PS Converter2/1
  Demux1/3 -> Simulink-PS Converter4/1
  Demux1/4 -> Simulink-PS Converter5/1
  Demux1/5 -> Simulink-PS Converter6/1
  Demux1/6 -> Simulink-PS Converter7/1
  Gain/1 -> Angular_vel_measured/1
  connections:
  Wheel and Axle/LConn1 -- Worm Gear/RConn1
  Mass/LConn1 -- Wheel and Axle/RConn1
  Motor & Drive (System Level)/RConn1 -- Converter (Three-Phase)/RConn2 -- DC Voltage Source/RConn1 -- Electrical Reference/LConn1 -- Solver Configuration/RConn1
  Motor & Drive (System Level)/RConn3 -- Mechanical Rotational Reference/LConn1
  Motor & Drive (System Level)/LConn3 -- Worm Gear/LConn1
  PS-Simulink Converter1/LConn1 -- Motor & Drive (System Level)/RConn2
  Motor & Drive (System Level)/LConn2 -- Simulink-PS Converter3/RConn1
  Simulink-PS Converter1/RConn1 -- Six-Pulse Gate Multiplexer/LConn1
  Simulink-PS Converter2/RConn1 -- Six-Pulse Gate Multiplexer/LConn2
  Simulink-PS Converter4/RConn1 -- Six-Pulse Gate Multiplexer/LConn3
  Simulink-PS Converter5/RConn1 -- Six-Pulse Gate Multiplexer/LConn4
  Simulink-PS Converter6/RConn1 -- Six-Pulse Gate Multiplexer/LConn5
  Simulink-PS Converter7/RConn1 -- Motor & Drive (System Level)/LConn4 -- Six-Pulse Gate Multiplexer/LConn6
  DC Voltage Source/LConn1 -- Converter (Three-Phase)/RConn1 -- Motor & Drive (System Level)/LConn1
  Converter (Three-Phase)/LConn1 -- Six-Pulse Gate Multiplexer/RConn1

== system PMSM_Hall_model/Inverter/Subsystem2/Subsystem ==
  Duty Cycle : Inport
  Gain1 : Gain  Gain=-1
  Gate_Inverter1 : Subsystem
  Gate_Lowside : Outport
  wires:
  Gate_Inverter1/1(Out1) -> Gate_Lowside/1
  Gain1/1 -> Gate_Inverter1/1(In1)
  Duty Cycle/1 -> Gain1/1

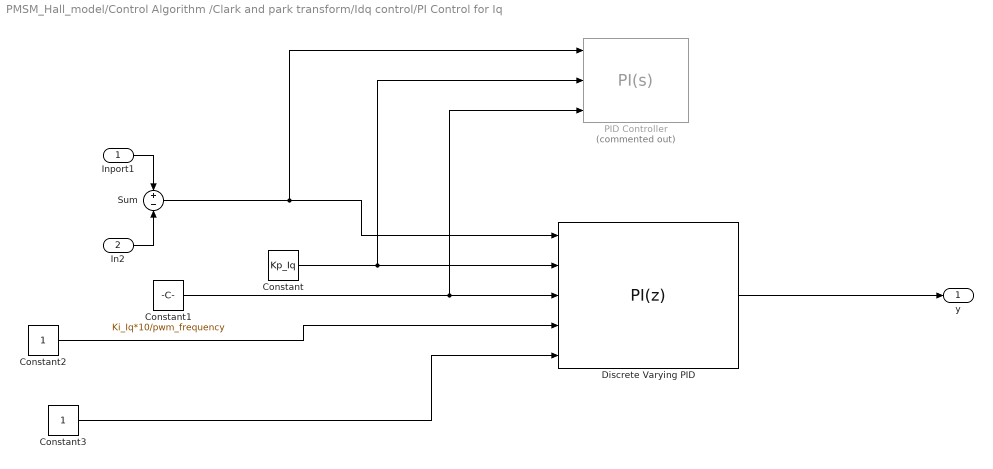
== system PMSM_Hall_model/Control Algorithm /Clark and park transform/Idq control/PI Control for Iq ==
  Inport1 : Inport
  In2 : Inport  Port=2
  Constant : Constant  Value=Kp_Iq
  Constant1 : Constant  Value=Ki_Iq*10/pwm_frequency
  Constant2 : Constant
  Constant3 : Constant
  Discrete Varying PID : slpidlib/PID Controller  Controller=PI  Form=Parallel  TimeDomain=Discrete-time  UseExternalTs=off  SampleTime=-1  IntegratorMethod=Forward Euler  FilterMethod=Forward Euler  ControllerParametersSource=external  P=1  I=1  UseKiTs=on  D=0  UseExternalDerivativeSource=off  N=100  UseFilter=off  TunerSelectOption=Transfer Function Based (PID Tuner App)  InitialConditionSource=external  InitialConditionForIntegrator=0  InitialConditionForFilter=0  DifferentiatorICPrevScaledInput=0  ExternalReset=level  TrackingMode=off  Kt=1  LimitOutput=on  SatLimitsSource=internal  UpperSaturationLimit=1  LowerSaturationLimit=-1  LinearizeAsGain=on  AntiWindupMode=clamping  Kb=1  LimitIntegrator=off  UpperIntegratorSaturationLimit=inf  LowerIntegratorSaturationLimit=-inf  POutMin=[]  POutMax=[]  IOutMin=[]  IOutMax=[]  DOutMin=[]  DOutMax=[]  NOutMin=[]  NOutMax=[]  SumOutMin=[]  SumOutMax=[]  SaturationOutMin=[]  SaturationOutMax=[]  PParamMin=[]  PParamMax=[]  IParamMin=[]  IParamMax=[]  DParamMin=[]  DParamMax=[]  NParamMin=[]  NParamMax=[]  KbParamMin=[]  KbParamMax=[]  KtParamMin=[]  KtParamMax=[]  KbOutMin=[]  KbOutMax=[]  KtOutMin=[]  KtOutMax=[]  IntegratorOutMin=[]  IntegratorOutMax=[]  FilterOutMin=[]  FilterOutMax=[]  SumI1OutMin=[]  SumI1OutMax=[]  SumI2OutMin=[]  SumI2OutMax=[]  SumI3OutMin=[]  SumI3OutMax=[]  SumI4OutMin=[]  SumI4OutMax=[]  SumDOutMin=[]  SumDOutMax=[]  DifferentiatorOutMin=[]  DifferentiatorOutMax=[]  FilterDiffOutCoefMin=[]  FilterDiffOutCoefMax=[]  ReciprocalOutMin=[]  ReciprocalOutMax=[]  SumDenOutMin=[]  SumDenOutMax=[]  SumNumOutMin=[]  SumNumOutMax=[]  DivideOutMin=[]  DivideOutMax=[]  UdiffTsProdOutMin=[]  UdiffTsProdOutMax=[]  NTsProdOutMin=[]  NTsProdOutMax=[]  UintegralTsProdOutMin=[]  UintegralTsProdOutMax=[]  UngainTsProdOutMin=[]  UngainTsProdOutMax=[]  ClampingZeroOutDataTypeStr=Inherit: Inherit via back propagation  ClampingZeroOutMin=[]  ClampingZeroOutMax=[]  FilterDenConstantOutDataTypeStr=Inherit: Inherit via back propagation  FilterDenConstantOutMin=[]  FilterDenConstantOutMax=[]  PCopyOutDataTypeStr=Inherit: Inherit via back propagation  PCopyOutMin=[]  PCopyOutMax=[]  NCopyOutDataTypeStr=Inherit: Inherit via back propagation  NCopyOutMin=[]  NCopyOutMax=[]  IntegratorContinuousStateAttributes=''  IntegratorStateMustResolveToSignalObject=off  IntegratorRTWStateStorageClass=Auto  FilterContinuousStateAttributes=''  FilterStateMustResolveToSignalObject=off  FilterRTWStateStorageClass=Auto  ParallelPVariant=ExternalParameters  IdealPVariant=Disabled  IVariant=ExternalParameters  DVariant=Disabled  IntegratorVariant=Discrete  SatVariant=Enabled  AWVariant=DiscClampingParallel  PCopyVariant=Disabled  TRVariant=Disabled  FdbkBlocksVariant=Forward  IdealPFdbkVariant=Disabled  SatFdbkVariant=Disabled  DerivativeFilterVariant=Disabled  NVariant=Disabled  NCopyVariant=Disabled_SignalSpec  FilterICVariant=Disabled  IntegratorICVariant=ExternalICs  ExternalResetVariant=ExternalReset  TRSumVariant=Passthrough  SumFdbkVariant=Disabled  SumVariant=Sum_PI  TsampFilterVariant=InternalTs  TsampNgainVariant=Passthrough  TsampIntegralVariant=Disabled_SignalSpec  ExternalSaturationOutDataTypeStr=Inherit: Same as second input  DerivativeSourceVariant=Disabled  PreIntVariant=InternalPreInt
      settings: LibrarySourceBlock=cstblocks/Linear Parameter Varying/Discrete Varying PID
  PID Controller : slpidlib/PID Controller  Commented=on  Controller=PI  Form=Parallel  TimeDomain=Continuous-time  UseExternalTs=off  SampleTime=-1  IntegratorMethod=Forward Euler  FilterMethod=Forward Euler  ControllerParametersSource=external  P=1  I=1  UseKiTs=on  D=0  UseExternalDerivativeSource=off  N=100  UseFilter=on  TunerSelectOption=Transfer Function Based (PID Tuner App)  ZeroCross=off  InitialConditionSource=internal  InitialConditionForIntegrator=0  InitialConditionForFilter=0  DifferentiatorICPrevScaledInput=0  ExternalReset=none  TrackingMode=off  Kt=1  LimitOutput=off  SatLimitsSource=internal  UpperSaturationLimit=inf  LowerSaturationLimit=-inf  LinearizeAsGain=on  AntiWindupMode=none  Kb=1  LimitIntegrator=off  UpperIntegratorSaturationLimit=inf  LowerIntegratorSaturationLimit=-inf  POutMin=[]  POutMax=[]  IOutMin=[]  IOutMax=[]  DOutMin=[]  DOutMax=[]  NOutMin=[]  NOutMax=[]  SumOutMin=[]  SumOutMax=[]  SaturationOutMin=[]  SaturationOutMax=[]  PParamMin=[]  PParamMax=[]  IParamMin=[]  IParamMax=[]  DParamMin=[]  DParamMax=[]  NParamMin=[]  NParamMax=[]  KbParamMin=[]  KbParamMax=[]  KtParamMin=[]  KtParamMax=[]  KbOutMin=[]  KbOutMax=[]  KtOutMin=[]  KtOutMax=[]  IntegratorOutMin=[]  IntegratorOutMax=[]  FilterOutMin=[]  FilterOutMax=[]  SumI1OutMin=[]  SumI1OutMax=[]  SumI2OutMin=[]  SumI2OutMax=[]  SumI3OutMin=[]  SumI3OutMax=[]  SumI4OutMin=[]  SumI4OutMax=[]  SumDOutMin=[]  SumDOutMax=[]  DifferentiatorOutMin=[]  DifferentiatorOutMax=[]  FilterDiffOutCoefMin=[]  FilterDiffOutCoefMax=[]  ReciprocalOutMin=[]  ReciprocalOutMax=[]  SumDenOutMin=[]  SumDenOutMax=[]  SumNumOutMin=[]  SumNumOutMax=[]  DivideOutMin=[]  DivideOutMax=[]  UdiffTsProdOutMin=[]  UdiffTsProdOutMax=[]  NTsProdOutMin=[]  NTsProdOutMax=[]  UintegralTsProdOutMin=[]  UintegralTsProdOutMax=[]  UngainTsProdOutMin=[]  UngainTsProdOutMax=[]  ClampingZeroOutDataTypeStr=Inherit: Inherit via back propagation  ClampingZeroOutMin=[]  ClampingZeroOutMax=[]  FilterDenConstantOutDataTypeStr=Inherit: Inherit via back propagation  FilterDenConstantOutMin=[]  FilterDenConstantOutMax=[]  PCopyOutDataTypeStr=Inherit: Inherit via back propagation  PCopyOutMin=[]  PCopyOutMax=[]  NCopyOutDataTypeStr=Inherit: Inherit via back propagation  NCopyOutMin=[]  NCopyOutMax=[]  IntegratorContinuousStateAttributes=''  IntegratorStateMustResolveToSignalObject=off  IntegratorRTWStateStorageClass=Auto  FilterContinuousStateAttributes=''  FilterStateMustResolveToSignalObject=off  FilterRTWStateStorageClass=Auto  ParallelPVariant=ExternalParameters  IdealPVariant=Disabled  IVariant=ExternalParameters  DVariant=Disabled  IntegratorVariant=Continuous  SatVariant=Disabled  AWVariant=Passthrough  PCopyVariant=Disabled  TRVariant=Disabled  FdbkBlocksVariant=Forward  IdealPFdbkVariant=Disabled  SatFdbkVariant=Disabled  DerivativeFilterVariant=Disabled  NVariant=Disabled  NCopyVariant=Disabled_SignalSpec  FilterICVariant=Disabled  IntegratorICVariant=InternalICs  ExternalResetVariant=Disabled  TRSumVariant=Passthrough  SumFdbkVariant=Disabled  SumVariant=Sum_PI  TsampFilterVariant=InternalTs  TsampNgainVariant=Passthrough  TsampIntegralVariant=Disabled_SignalSpec  ExternalSaturationOutDataTypeStr=Inherit: Same as second input  DerivativeSourceVariant=Disabled  PreIntVariant=InternalPreInt
  Sum : Sum  Inputs=+-
  y : Outport
  wires:
  Constant/1 -> PID Controller/2, Discrete Varying PID/2
  Constant1/1 -> PID Controller/3, Discrete Varying PID/3
  In2/1 -> Sum/2
  Inport1/1 -> Sum/1
  Sum/1 -> PID Controller/1, Discrete Varying PID/1
  Constant2/1 -> Discrete Varying PID/4
  Constant3/1 -> Discrete Varying PID/5
  Discrete Varying PID/1 -> y/1

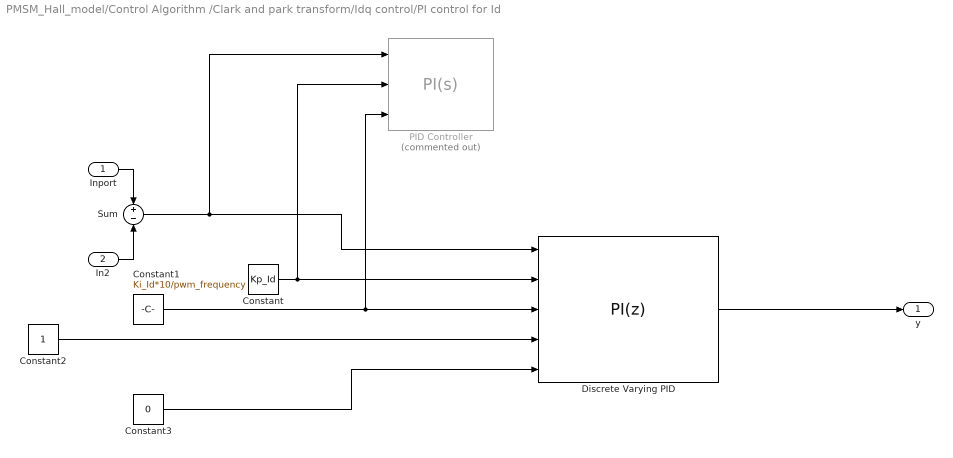
== system PMSM_Hall_model/Control Algorithm /Clark and park transform/Idq control/PI control for Id ==
  Inport : Inport
  In2 : Inport  Port=2
  Constant : Constant  Value=Kp_Id
  Constant1 : Constant  Value=Ki_Id*10/pwm_frequency
  Constant2 : Constant
  Constant3 : Constant  Value=0
  Discrete Varying PID : slpidlib/PID Controller  Controller=PI  Form=Parallel  TimeDomain=Discrete-time  UseExternalTs=off  SampleTime=-1  IntegratorMethod=Forward Euler  FilterMethod=Forward Euler  ControllerParametersSource=external  P=1  I=1  UseKiTs=on  D=0  UseExternalDerivativeSource=off  N=100  UseFilter=off  TunerSelectOption=Transfer Function Based (PID Tuner App)  InitialConditionSource=external  InitialConditionForIntegrator=0  InitialConditionForFilter=0  DifferentiatorICPrevScaledInput=0  ExternalReset=level  TrackingMode=off  Kt=1  LimitOutput=on  SatLimitsSource=internal  UpperSaturationLimit=1  LowerSaturationLimit=-1  LinearizeAsGain=on  AntiWindupMode=clamping  Kb=1  LimitIntegrator=off  UpperIntegratorSaturationLimit=inf  LowerIntegratorSaturationLimit=-inf  POutMin=[]  POutMax=[]  IOutMin=[]  IOutMax=[]  DOutMin=[]  DOutMax=[]  NOutMin=[]  NOutMax=[]  SumOutMin=[]  SumOutMax=[]  SaturationOutMin=[]  SaturationOutMax=[]  PParamMin=[]  PParamMax=[]  IParamMin=[]  IParamMax=[]  DParamMin=[]  DParamMax=[]  NParamMin=[]  NParamMax=[]  KbParamMin=[]  KbParamMax=[]  KtParamMin=[]  KtParamMax=[]  KbOutMin=[]  KbOutMax=[]  KtOutMin=[]  KtOutMax=[]  IntegratorOutMin=[]  IntegratorOutMax=[]  FilterOutMin=[]  FilterOutMax=[]  SumI1OutMin=[]  SumI1OutMax=[]  SumI2OutMin=[]  SumI2OutMax=[]  SumI3OutMin=[]  SumI3OutMax=[]  SumI4OutMin=[]  SumI4OutMax=[]  SumDOutMin=[]  SumDOutMax=[]  DifferentiatorOutMin=[]  DifferentiatorOutMax=[]  FilterDiffOutCoefMin=[]  FilterDiffOutCoefMax=[]  ReciprocalOutMin=[]  ReciprocalOutMax=[]  SumDenOutMin=[]  SumDenOutMax=[]  SumNumOutMin=[]  SumNumOutMax=[]  DivideOutMin=[]  DivideOutMax=[]  UdiffTsProdOutMin=[]  UdiffTsProdOutMax=[]  NTsProdOutMin=[]  NTsProdOutMax=[]  UintegralTsProdOutMin=[]  UintegralTsProdOutMax=[]  UngainTsProdOutMin=[]  UngainTsProdOutMax=[]  ClampingZeroOutDataTypeStr=Inherit: Inherit via back propagation  ClampingZeroOutMin=[]  ClampingZeroOutMax=[]  FilterDenConstantOutDataTypeStr=Inherit: Inherit via back propagation  FilterDenConstantOutMin=[]  FilterDenConstantOutMax=[]  PCopyOutDataTypeStr=Inherit: Inherit via back propagation  PCopyOutMin=[]  PCopyOutMax=[]  NCopyOutDataTypeStr=Inherit: Inherit via back propagation  NCopyOutMin=[]  NCopyOutMax=[]  IntegratorContinuousStateAttributes=''  IntegratorStateMustResolveToSignalObject=off  IntegratorRTWStateStorageClass=Auto  FilterContinuousStateAttributes=''  FilterStateMustResolveToSignalObject=off  FilterRTWStateStorageClass=Auto  ParallelPVariant=ExternalParameters  IdealPVariant=Disabled  IVariant=ExternalParameters  DVariant=Disabled  IntegratorVariant=Discrete  SatVariant=Enabled  AWVariant=DiscClampingParallel  PCopyVariant=Disabled  TRVariant=Disabled  FdbkBlocksVariant=Forward  IdealPFdbkVariant=Disabled  SatFdbkVariant=Disabled  DerivativeFilterVariant=Disabled  NVariant=Disabled  NCopyVariant=Disabled_SignalSpec  FilterICVariant=Disabled  IntegratorICVariant=ExternalICs  ExternalResetVariant=ExternalReset  TRSumVariant=Passthrough  SumFdbkVariant=Disabled  SumVariant=Sum_PI  TsampFilterVariant=InternalTs  TsampNgainVariant=Passthrough  TsampIntegralVariant=Disabled_SignalSpec  ExternalSaturationOutDataTypeStr=Inherit: Same as second input  DerivativeSourceVariant=Disabled  PreIntVariant=InternalPreInt
      settings: LibrarySourceBlock=cstblocks/Linear Parameter Varying/Discrete Varying PID
  PID Controller : slpidlib/PID Controller  Commented=on  Controller=PI  Form=Parallel  TimeDomain=Continuous-time  UseExternalTs=off  SampleTime=-1  IntegratorMethod=Forward Euler  FilterMethod=Forward Euler  ControllerParametersSource=external  P=1  I=1  UseKiTs=on  D=0  UseExternalDerivativeSource=off  N=100  UseFilter=on  TunerSelectOption=Transfer Function Based (PID Tuner App)  InitialConditionSource=internal  InitialConditionForIntegrator=0  InitialConditionForFilter=0  DifferentiatorICPrevScaledInput=0  ExternalReset=none  TrackingMode=off  Kt=1  LimitOutput=off  SatLimitsSource=internal  UpperSaturationLimit=inf  LowerSaturationLimit=-inf  LinearizeAsGain=on  AntiWindupMode=none  Kb=1  LimitIntegrator=off  UpperIntegratorSaturationLimit=inf  LowerIntegratorSaturationLimit=-inf  POutMin=[]  POutMax=[]  IOutMin=[]  IOutMax=[]  DOutMin=[]  DOutMax=[]  NOutMin=[]  NOutMax=[]  SumOutMin=[]  SumOutMax=[]  SaturationOutMin=[]  SaturationOutMax=[]  PParamMin=[]  PParamMax=[]  IParamMin=[]  IParamMax=[]  DParamMin=[]  DParamMax=[]  NParamMin=[]  NParamMax=[]  KbParamMin=[]  KbParamMax=[]  KtParamMin=[]  KtParamMax=[]  KbOutMin=[]  KbOutMax=[]  KtOutMin=[]  KtOutMax=[]  IntegratorOutMin=[]  IntegratorOutMax=[]  FilterOutMin=[]  FilterOutMax=[]  SumI1OutMin=[]  SumI1OutMax=[]  SumI2OutMin=[]  SumI2OutMax=[]  SumI3OutMin=[]  SumI3OutMax=[]  SumI4OutMin=[]  SumI4OutMax=[]  SumDOutMin=[]  SumDOutMax=[]  DifferentiatorOutMin=[]  DifferentiatorOutMax=[]  FilterDiffOutCoefMin=[]  FilterDiffOutCoefMax=[]  ReciprocalOutMin=[]  ReciprocalOutMax=[]  SumDenOutMin=[]  SumDenOutMax=[]  SumNumOutMin=[]  SumNumOutMax=[]  DivideOutMin=[]  DivideOutMax=[]  UdiffTsProdOutMin=[]  UdiffTsProdOutMax=[]  NTsProdOutMin=[]  NTsProdOutMax=[]  UintegralTsProdOutMin=[]  UintegralTsProdOutMax=[]  UngainTsProdOutMin=[]  UngainTsProdOutMax=[]  ClampingZeroOutDataTypeStr=Inherit: Inherit via back propagation  ClampingZeroOutMin=[]  ClampingZeroOutMax=[]  FilterDenConstantOutDataTypeStr=Inherit: Inherit via back propagation  FilterDenConstantOutMin=[]  FilterDenConstantOutMax=[]  PCopyOutDataTypeStr=Inherit: Inherit via back propagation  PCopyOutMin=[]  PCopyOutMax=[]  NCopyOutDataTypeStr=Inherit: Inherit via back propagation  NCopyOutMin=[]  NCopyOutMax=[]  IntegratorContinuousStateAttributes=''  IntegratorStateMustResolveToSignalObject=off  IntegratorRTWStateStorageClass=Auto  FilterContinuousStateAttributes=''  FilterStateMustResolveToSignalObject=off  FilterRTWStateStorageClass=Auto  ParallelPVariant=ExternalParameters  IdealPVariant=Disabled  IVariant=ExternalParameters  DVariant=Disabled  IntegratorVariant=Continuous  SatVariant=Disabled  AWVariant=Passthrough  PCopyVariant=Disabled  TRVariant=Disabled  FdbkBlocksVariant=Forward  IdealPFdbkVariant=Disabled  SatFdbkVariant=Disabled  DerivativeFilterVariant=Disabled  NVariant=Disabled  NCopyVariant=Disabled_SignalSpec  FilterICVariant=Disabled  IntegratorICVariant=InternalICs  ExternalResetVariant=Disabled  TRSumVariant=Passthrough  SumFdbkVariant=Disabled  SumVariant=Sum_PI  TsampFilterVariant=InternalTs  TsampNgainVariant=Passthrough  TsampIntegralVariant=Disabled_SignalSpec  ExternalSaturationOutDataTypeStr=Inherit: Same as second input  DerivativeSourceVariant=Disabled  PreIntVariant=InternalPreInt
  Sum : Sum  Inputs=+-
  y : Outport
  wires:
  Constant/1 -> PID Controller/2, Discrete Varying PID/2
  Sum/1 -> PID Controller/1, Discrete Varying PID/1
  In2/1 -> Sum/2
  Constant1/1 -> PID Controller/3, Discrete Varying PID/3
  Inport/1 -> Sum/1
  Constant2/1 -> Discrete Varying PID/4
  Constant3/1 -> Discrete Varying PID/5
  Discrete Varying PID/1 -> y/1

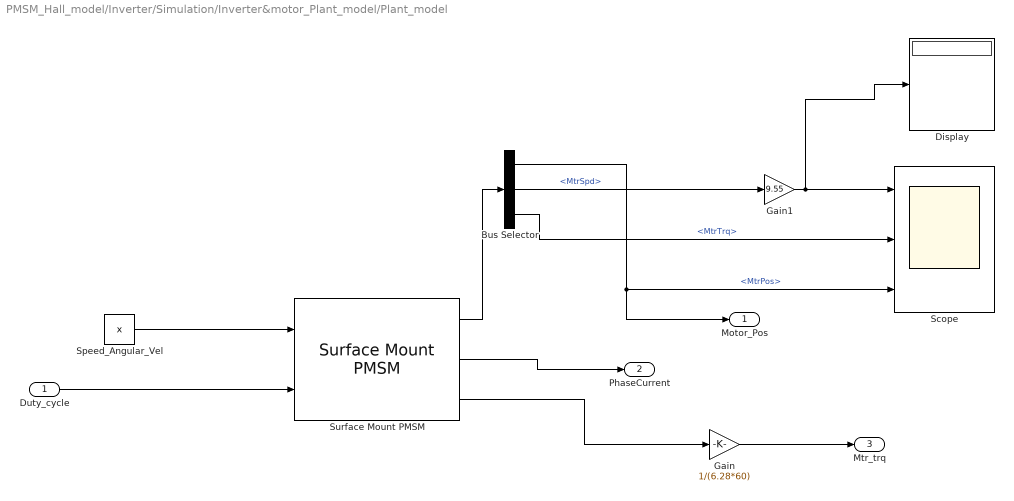
== system PMSM_Hall_model/Inverter/Simulation/Inverter&motor_Plant_model/Plant_model ==
  Duty_cycle : Inport
  Bus Selector : BusSelector  OutputSignals=MtrPos,MtrSpd,MtrTrq
  Display : Display
  Gain : Gain  Gain=1/(6.28*60)
  Gain1 : Gain  Gain=9.55
  Scope : Scope  NumInputPorts=3
      settings: ActiveDisplayYMinimum=-2.2231896464001126  ActiveDisplayYMaximum=1.4698219306560629  DataLoggingVariableName=ScopeData6
  Speed_Angular_Vel : Constant  Value=x
  Surface Mount PMSM : autolibpmsmexterior/Surface Mount PMSM  port_config=Speed  sim_type=Continuous  Ts=0.001  FilePath=E:\Sandbox\Bauto\Work\surfacepmsm_motordata.m  P=motor_polepairs  Rs=R_s  Ldq_=Ld  KConstText=Permanent flux linkage constant (lambda_pm):  lambda_pm=flux_linkage  Ke=159.9771  Kt=0.035  mechanical=[J,Damping_viscous,B]  idq0=[0 0]  theta_init=0  omega_init=0  KConst=0.1194  lambda_pm_calc=0.1194  RefBlkName='autolibpmsmexterior/Surface Mount PMSM'  aMode=1  Ldq="[0.0003752   0.0003752]"
      settings: LibrarySourceBlock=autolibemachines/Surface Mount PMSM
  Motor_Pos : Outport
  PhaseCurrent : Outport  Port=2
  Mtr_trq : Outport  Port=3
  wires:
  Duty_cycle/1 -> Surface Mount PMSM/2
  Surface Mount PMSM/2 -> PhaseCurrent/1
  Surface Mount PMSM/1 -> Bus Selector/1
  Bus Selector/1 -> Scope/3, Motor_Pos/1  "<MtrPos>"
  Bus Selector/2 -> Gain1/1  "<MtrSpd>"
  Gain1/1 -> Display/1, Scope/1
  Gain/1 -> Mtr_trq/1
  Bus Selector/3 -> Scope/2  "<MtrTrq>"
  Surface Mount PMSM/3 -> Gain/1
  Speed_Angular_Vel/1 -> Surface Mount PMSM/1

== system PMSM_Hall_model/Inverter/Subsystem2/Subsystem/Gate_Inverter1 ==
  In1 : Inport
  Add : Sum
  Constant1 : Constant
  Gain5 : Gain
  Out1 : Outport
  wires:
  Constant1/1 -> Add/2
  Add/1 -> Gain5/1
  Gain5/1 -> Out1/1
  In1/1 -> Add/1
